simulink model "dieu_che_PWM"  (R2019a)
settings: Solver=VariableStepAuto  StartTime=0.0  StopTime=0.001  RelTol=1e-3
settings Model: Creator=FPTSHOP  LastModifiedBy=Phong

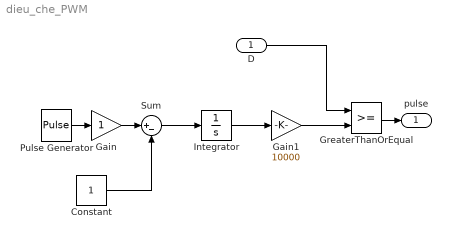
== system dieu_che_PWM ==
  D : Inport
  Constant : Constant
  Gain : Gain
  Gain1 : Gain  Gain=10000
  GreaterThanOrEqual : RelationalOperator  OutDataTypeStr=boolean  RndMeth=Simplest
  Integrator : Integrator
  Pulse Generator : DiscretePulseGenerator  PulseType=Time based  Amplitude=2  Period=1/5000  PulseWidth=50
  Sum : Sum  Inputs=|+-
  "pulse " : Outport
  wires:
  Gain1/1 -> GreaterThanOrEqual/2
  Constant/1 -> Sum/2
  Gain/1 -> Sum/1
  Integrator/1 -> Gain1/1
  Sum/1 -> Integrator/1
  GreaterThanOrEqual/1 -> "pulse "/1
  Pulse Generator/1 -> Gain/1
  D/1 -> GreaterThanOrEqual/1
